simulink model "Drone_simulation"  (R2025b)
settings: Solver=VariableStepAuto  StartTime=0.0  StopTime=15.0  RelTol=1e-3
libraries: slctrl_adaptive x1
settings Model: Creator=Shivani  LastModifiedBy=Shivani

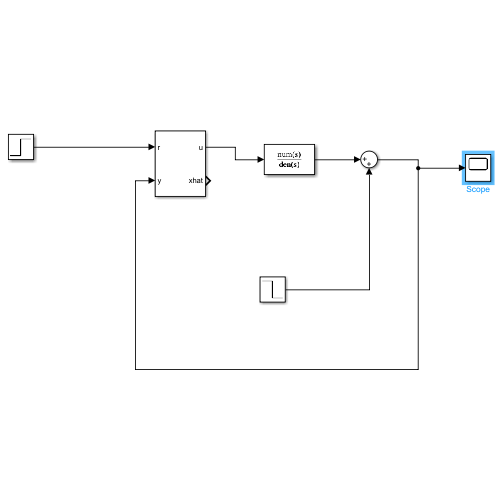
[thumbnail: Simulink's stored preview of the top-level diagram]
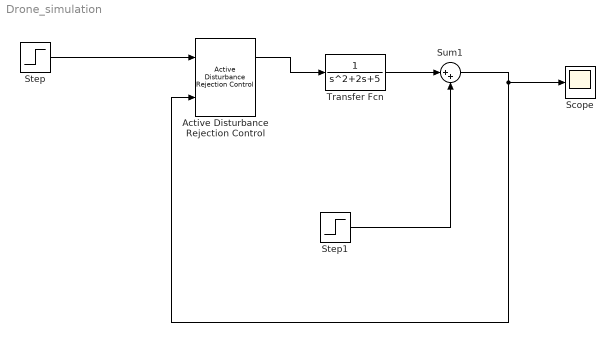
== system Drone_simulation ==
  Active Disturbance Rejection Control : slctrl_adaptive/Active Disturbance Rejection Control  time_domain=continuous-time  Ts=0.01  model_type=second-order  b0=1  wc=10  wo=100  x0=0  ulim_checkbox=off  umax=inf  umin=-inf  xhat_checkbox=on
      settings: LibrarySourceBlock=slctrlblks/Adaptive Control/Active Disturbance Rejection Control
  Scope : Scope
      settings: ActiveDisplayYMinimum=-0.14069468215465619  ActiveDisplayYMaximum=1.266252139391906
  Step : Step  Time=0  SampleTime=0
  Step1 : Step  Time=5  After=-0.5  SampleTime=0
  Sum1 : Sum  Inputs=|++
  Transfer Fcn : TransferFcn  Denominator=[1 2 5 ]
  wires:
  Step/1 -> Active Disturbance Rejection Control/1
  Active Disturbance Rejection Control/1 -> Transfer Fcn/1
  Transfer Fcn/1 -> Sum1/1
  Sum1/1 -> Active Disturbance Rejection Control/2, Scope/1
  Step1/1 -> Sum1/2
